simulink model "RDA_simulink_tes"  (R2020b)
settings: Solver=FixedStepAuto  StartTime=0.0  StopTime=10.0  FixedStep=0.001  RelTol=1e-3
InitFcn:
  | coder.extrinsic('pnet.mexw64')
  | recorderip = '127.0.0.1';
  | stat = 0;
  | con = 0;
  | tryheader = false;
  | % persistent props
  | % props = struct('channelCount',[uint32(0)],'samplingInterval',[0],'resolutions',[zeros(1,34)],'channelNames',[0]);
  | lastBlock = uint32(-1);
  | data1s = single(zeros(1));
  | coder.varsize('data1s')
  | EEGData = single(zeros(34, 680 / 34));
  | EEGdata32 = single(zeros(1, 20));
  |     % Establish connection to BrainVision Recorder Software 32Bit RDA-Port
  |     % (use 51234 to connect with 16Bit Port)
  | con = pnet('tcpconnect', recorderip, 51244);
  | 
  |     % Check established connection and display a message
  | stat = pnet(con,'status');
  | if stat > 0
  |     disp('connection established');
  | end
StopFcn:
  |     pnet('closeall');
  |     disp('connection closed');
libraries: sldrtlib x1
settings Model: Creator=Wacom hrg  LastModifiedBy=Wacom hrg

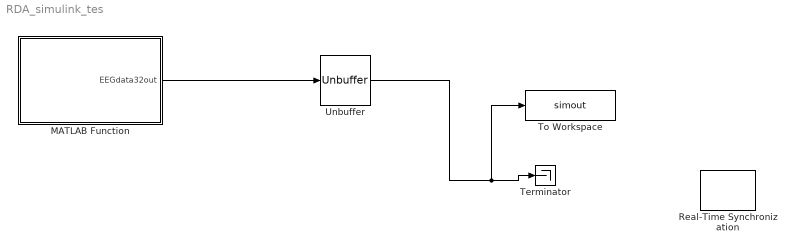
== system RDA_simulink_tes ==
  MATLAB Function : MATLAB Function  TreatAsAtomicUnit=on
  Real-Time Synchronization : sldrtlib/Real-Time Synchronization  SampleTime=0.1  MaxMissedTicks=10  ShowMissedTicks=off  YieldWhenWaiting=off
  Terminator : Terminator
  To Workspace : ToWorkspace  VariableName=simout  SaveFormat=Timeseries  SampleTime=-1
  Unbuffer : Unbuffer
  wires:
  Unbuffer/1 -> To Workspace/1, Terminator/1
  MATLAB Function/1(EEGdata32out) -> Unbuffer/1

== matlab function RDA_simulink_tes/MATLAB Function ==
  data: EEGdata32out output; tryheader parameter; con parameter; lastBlock parameter; data1s parameter; EEGData parameter
%% ***********************************************************************   
% Simple MATLAB RDA Client
%
% Demonstration file for implementing a simple MATLAB client for the
% RDA tcpip interface of the BrainVision Recorder.
% It reads all information of the recorded EEG,
% prints EEG and marker information to the
% MATLAB console and calculates and prints the average power every second.
%
%
% Brain Products GmbH 
% Gilching/Freiburg, Germany
% www.brainproducts.com
%
%
% This RDA Client uses version 2.x of the tcp/udp/ip Toolbox by
% Peter Rydesäter which can be downloaded from the Mathworks website
%
% 

%% ***********************************************************************   
% Main RDA Client function
function EEGdata32out  =  RDA(tryheader, con, lastBlock, data1s, EEGData)
    coder.extrinsic('pnet')
%     pause(1)
    % Change for individual recorder host
%     recorderip = '127.0.0.1';
%     stat = 0;
%     con = 0;
% %     tryheader = blanks(24); 
%     tryheader = false; 
%     coder.varsize('tryheader')
%     props = struct('channelCount',[uint32(0)],'samplingInterval',[0],'resolutions',[zeros(1,34)],'channelNames',[0]);
%     lastBlock = uint32(-1); 
%     data1s = single(zeros(0)); 
%     EEGdata = single(zeros(34, 680 / 34));
%     % Establish connection to BrainVision Recorder Software 32Bit RDA-Port
%     % (use 51234 to connect with 16Bit Port)
%     con = pnet('tcpconnect', recorderip, 51244);
%     
%     % Check established connection and display a message
%     stat = pnet(con,'status');
%     if stat > 0
%         disp('connection established');
%     end
    persistent props
    if isempty(props)
       props = struct('channelCount',[uint32(0)],'samplingInterval',[0],'resolutions',[zeros(1,34)],'channelNames',[0]);
    end
    persistent EEGdata32
    if isempty(EEGdata32)
            EEGdata32 = single(NaN(1, 20))';
    end 
    persistent counter
    if isempty(counter)
        counter = 1;
    end
    % --- Main reading loop ---
    header_size = 24;
        % check for existing data in socket buffer
    tryheader = ~isempty(pnet(con, 'read', header_size, 'byte', 'network', 'view', 'noblock'));
%     disp(tryheader)
    if tryheader%~isempty(tryheader)
        % Read header of RDA message
        hdr = ReadHeader(con);
        % Perform some action depending of the type of the data package
%         disp('hdrtype')
%         disp(hdr.type)
        switch hdr.type
            case 1       % Start, Setup information like EEG properties
                disp('Start');
                % Read and display EEG properties
                

                props = ReadStartMessage(con, hdr);
                disp(props);

                % Reset block counter to check overflows
                lastBlock = uint32(-1);

                % set data buffer to empty
                data1s = single(zeros(0));

            case 4       % 32Bit Data block
                % Read data and markers from message
%                         disp('case4')
%                 disp(props)
                [datahdr, data, markers] = ReadDataMessage(con, hdr, props);
%                         disp('reading')

                % check tcpip buffer overflow
                if lastBlock ~= uint32(-1) && datahdr.block > lastBlock + 1
                    disp(['******* Overflow with ' int2str(datahdr.block - lastBlock) ' blocks ******']);
                end
                lastBlock = datahdr.block;
%                         disp('lastblock')
                disp(datahdr)
                % print marker info to MATLAB console
                if datahdr.markerCount > 0
                    for m = 1:datahdr.markerCount
                        disp(markers(m));
                    end    
                end

                % Process EEG data, 
                % in this case extract last recorded second,
%                 disp(size(data))
                EEGData = reshape(data, props.channelCount, length(data) / props.channelCount);
                EEGdata32 = EEGData(2,1:20)';
%                     disp('EEG')
%                     disp(EEGData)
%                     data1s = [data1s EEGData];
             
                dims = size(data1s);
                if dims(2) > 1000000 / props.samplingInterval
%                     data1s = data1s(:, dims(2) - 1000000 / props.samplingInterval : dims(2));
                    avg = mean(mean(data1s.*data1s));
%                             disp(['Average power: ' num2str(avg)]);
                    % set data buffer to empty for next full second
%                     data1s = single(zeros(0));
                end
            case 3       % Stop message   
                disp('Stop');
                        data = pnet(con, 'read', hdr.size - header_size);
%                 data = 0;
                finish = true;

            otherwise    % ignore all unknown types, but read the package from buffer 
                        data = pnet(con, 'read', hdr.size - header_size);
%                 data = 0;
%                 disp('other')
                EEGdata32 = single(NaN(1,20)');
        end
    end
    EEGdata32out =EEGdata32;
end
    
    

%% ***********************************************************************
% Read the message header
function hdr = ReadHeader(con)
    % con    tcpip connection object
    coder.extrinsic('pnet')
    % define a struct for the header
    hdr = struct('uid',blanks(16),'size',[uint32(0)],'type',[uint32(0)]);
%     coder.varsize('size')
%     coder.varsize('type')

    % read id, size and type of the message
    % swapbytes is important for correct byte order of MATLAB variables
    % pnet behaves somehow strange with byte order option
    hdr.uid = pnet(con,'read', 16);
    hdr.size = swapbytes(pnet(con,'read', 1, 'uint32', 'network'));
    hdr.type = swapbytes(pnet(con,'read', 1, 'uint32', 'network'));

end

%% ***********************************************************************   
% Read the start message
function props = ReadStartMessage(con, hdr)
    % con    tcpip connection object    
    % hdr    message header
    % props  returned eeg properties
    coder.extrinsic('pnet')
    % define a struct for the EEG properties
    props = struct('channelCount',zeros(1,'uint32'),'samplingInterval',[0],'resolutions',[zeros(1,34)],'channelNames',[0]);
%     coder.varsize('channelCount')
%     coder.varsize('samplingInterval')
%     coder.varsize('resolutions')

    % read EEG properties
    props.channelCount = swapbytes(pnet(con,'read', 1, 'uint32', 'network'));
    props.samplingInterval = swapbytes(pnet(con,'read', 1, 'double', 'network'));
    props.resolutions = swapbytes(pnet(con,'read', props.channelCount, 'double', 'network'));
    allChannelNames = pnet(con,'read', hdr.size - 36 - props.channelCount * 8);
    props.channelNames = 0;% SplitChannelNames(allChannelNames);
end
    
%% ***********************************************************************   
% Read a data message
function [datahdr, data, markers] = ReadDataMessage(con, hdr, props)
    % con       tcpip connection object    
    % hdr       message header
    % props     eeg properties
    % datahdr   data header with information on datalength and number of markers
    % data      data as one dimensional arry
    % markers   markers as array of marker structs
    coder.extrinsic('pnet')
    % Define data header struct and read data header
    datahdr = struct('block',[uint32(0)],'points',[uint32(0)],'markerCount',[uint32(0)]);
%     coder.varsize('block')
%     coder.varsize('points')
%     coder.varsize('markerCount')

    datahdr.block = swapbytes(pnet(con,'read', 1, 'uint32', 'network'));
    datahdr.points = swapbytes(pnet(con,'read', 1, 'uint32', 'network'));
    datahdr.markerCount = swapbytes(pnet(con,'read', 1, 'uint32', 'network'));
%     disp('datahdr')
%     disp(datahdr)
%     disp(props)
    data = single(zeros(680));
    coder.varsize('data')
    % Read data in float format
    data = swapbytes(pnet(con,'read', props.channelCount * datahdr.points, 'single', 'network')); %props.channelCount datahdr.points
%     disp(data)
    % Define markers struct and read markers
    markers = struct('size',[],'position',[],'points',[],'channel',[],'type',[],'description',[]);
    for m = 1:datahdr.markerCount
        disp('Marker')
        marker = struct('size',[],'position',[],'points',[],'channel',[],'type',[],'description',[]);

        % Read integer information of markers
        marker.size = swapbytes(pnet(con,'read', 1, 'uint32', 'network'));
        marker.position = swapbytes(pnet(con,'read', 1, 'uint32', 'network'));
        marker.points = swapbytes(pnet(con,'read', 1, 'uint32', 'network'));
        marker.channel = swapbytes(pnet(con,'read', 1, 'int32', 'network'));

        % type and description of markers are zero-terminated char arrays
        % of unknown length
        c = zeros(1,1);
% NEED TO CHECK WHETHER WE CAN LEAVE THIS UNCOMMETED
%         c = pnet(con,'read', 1);
        while c ~= 0
%             marker.type = [marker.type c];
            c = pnet(con,'read', 1);
        end
% 
        c = pnet(con,'read', 1);
        while c ~= 0
%             marker.description = [marker.description c];
            c = pnet(con,'read', 1);
        end
    end
%         
%         % Add marker to array
%         markers(m) = marker;  

end

    
%% ***********************************************************************   
% Helper function for channel name splitting, used by function
% ReadStartMessage for extraction of channel names
function channelNames = SplitChannelNames(allChannelNames)
    % allChannelNames   all channel names together in an array of char
    % channelNames      channel names splitted in a cell array of strings

    % cell array to return
    channelNames = cell(1,34);
    
    % helper for actual name in loop
    name = [];
    namecount = 1;
    % loop over all chars in array
    for i = 1:length(allChannelNames)
        if allChannelNames(i) ~= 0
            % if not a terminating zero, add char to actual name
            name = [name allChannelNames(i)];
        else
            % add name to cell array and clear helper for reading next name
            channelNames{namecount} = name;
            name = [];
            namecount = namecount +1; 
        end
    end
end
